simulink model "SIMULINK_flexible_joint"  (R2024b)
settings: Solver=ode45  StartTime=0.0  StopTime=100  RelTol=1e-3  EnableMultiTasking=on
undefined symbols (not defined in the file): cix1, cix2, cix3, cix4, g, hcm, Jh, Jl, Kg, Km, Ks, Kz, Kzi, m, pert, Rm
libraries: simulink x1
settings Model: Creator=AP  LastModifiedBy=J Ferb
settings SolverCC: AlgebraicLoopSolver=TrustRegion
settings DataIOCC: LimitDataPoints=on  SaveFormat=Array  SignalLoggingSaveFormat=ModelDataLogs  ReturnWorkspaceOutputs=off
settings OptimizationCC: ExpressionDepthLimit=2147483647  InitFltsAndDblsToZero=on  LifeSpan=inf
settings DebuggingCC: SaveWithParameterizedLinksMsg=none  UnderspecifiedInitializationDetection=Classic  MergeDetectMultiDrivingBlocksExec=none  FcnCallInpInsideContextMsg=warning  UnconnectedInputMsg=warning  UnconnectedOutputMsg=warning  UnconnectedLineMsg=warning  StateNameClashWarn=warning  SFUnexpectedBacktrackingDiag=warning  SFNoUnconditionalDefaultTransitionDiag=warning  SFExecutionAtInitializationDiag=none  ArithmeticOperatorsInVariantConditions=warning
settings HardwareCC: ProdBitPerPointer=32  ProdBitPerSizeT=32  ProdBitPerPtrDiffT=32  ProdLargestAtomicFloat=None  ProdIntDivRoundTo=Undefined  ProdEndianess=Unspecified  ProdWordSize=32  ProdHWDeviceType=32-bit Generic
settings ModelReferenceCC: EnableRefExpFcnMdlSchedulingChecks=on  PropagateSignalLabelsOutOfModel=off
settings SFSimCC: SimParseCustomCode=off
settings RTWCC: GPUComputeCapability=3.5
settings CodeAppCC: StateflowObjectComments=on
settings GRTTargetCC: TargetFcnLib=ansi_tfl_tmw.mat  TargetLangStandard=C89/C90 (ANSI)  CombineOutputUpdateFcns=off  GRTInterface=on
settings ConfigComp: CovMetricSettings=dw  CovSaveCumulativeToWorkspaceVar=on  CovSaveSingleToWorkspaceVar=on

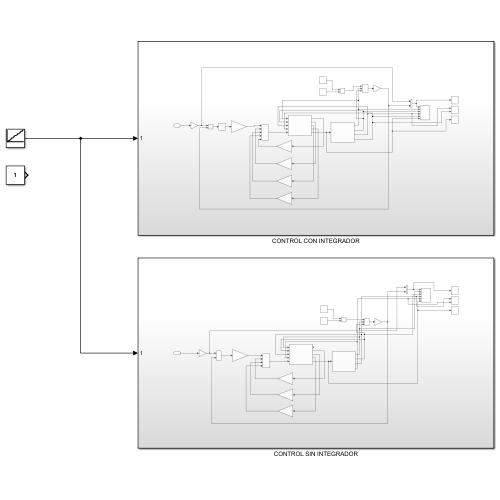
[thumbnail: Simulink's stored preview of the top-level diagram]
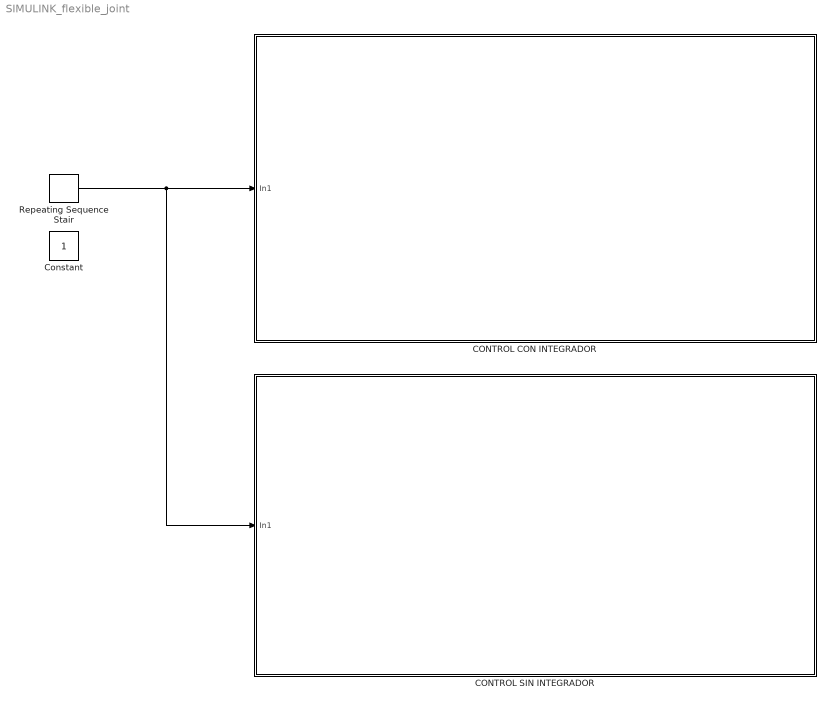
== system SIMULINK_flexible_joint ==
  CONTROL CON INTEGRADOR : Subsystem
  CONTROL SIN INTEGRADOR : Subsystem
  Constant : Constant
  Repeating Sequence Stair : simulink/Sources/Repeating Sequence Stair  OutValues=[0 0.02 0.04 0.06 0.08 0.1 0.12 0.14 0.16 0.18 0.2].'*1  tsamp=4  OutMin=[]  OutMax=[]  OutDataTypeStr=float('double')  OutputDataTypeScalingMode=Specify via dialog  OutDataType=float('double')  ConRadixGroup=Best Precision: Vector-wise  OutScaling=2^-12
  wires:
  Repeating Sequence Stair/1 -> CONTROL SIN INTEGRADOR/1(In1), CONTROL CON INTEGRADOR/1(In1)

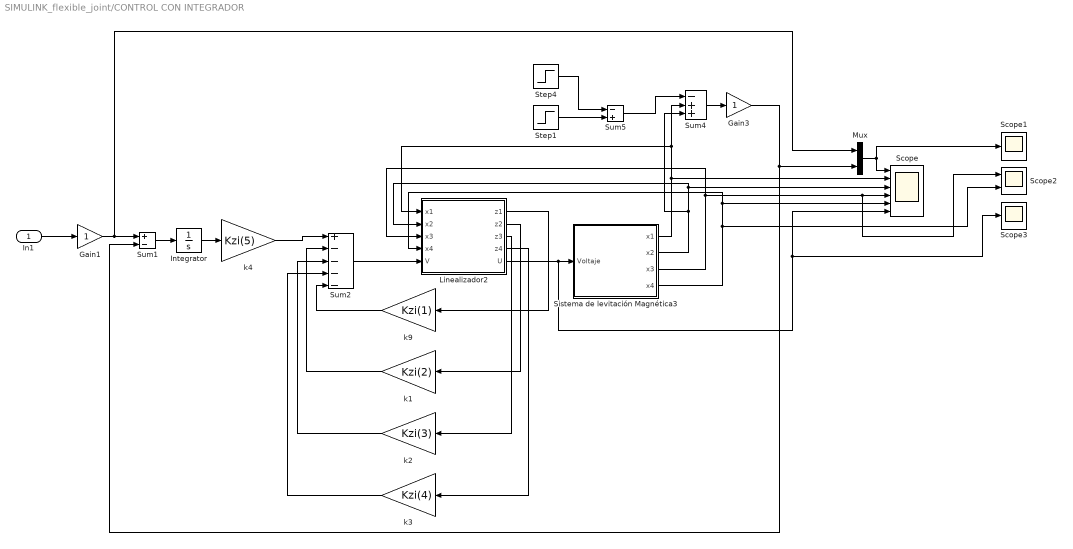
== system SIMULINK_flexible_joint/CONTROL CON INTEGRADOR ==
  In1 : Inport
  Gain1 : Gain
  Gain3 : Gain
  Integrator : Integrator
  Linealizador2 : Subsystem
  Mux : Mux  Inputs=2
  Scope : Scope  NumInputPorts=6
  Scope1 : Scope
  Scope2 : Scope  NumInputPorts=2
  Scope3 : Scope
  Sistema de levitación Magnética3 : Subsystem
  Step1 : Step  Time=5  After=pert  SampleTime=0
  Step4 : Step  Time=5.1  After=pert  SampleTime=0
  Sum1 : Sum  Inputs=+-
  Sum2 : Sum  Inputs=+----
  Sum4 : Sum  Inputs=-++
  Sum5 : Sum  Inputs=-+
  k1 : Gain  Gain=Kzi(2)
  k2 : Gain  Gain=Kzi(3)
  k3 : Gain  Gain=Kzi(4)
  k4 : Gain  Gain=Kzi(5)
  k9 : Gain  Gain=Kzi(1)
  wires:
  Sistema de levitación Magnética3/4(x4) -> Scope/5, Linealizador2/4(x4), Scope2/2
  Linealizador2/1(z1) -> k9/1
  Sum4/1 -> Gain3/1
  Sistema de levitación Magnética3/1(x1) -> Sum4/2, Linealizador2/1(x1), Scope/2
  k3/1 -> Sum2/4
  Linealizador2/4(z4) -> k3/1
  k1/1 -> Sum2/2
  k2/1 -> Sum2/3
  In1/1 -> Gain1/1
  Linealizador2/3(z3) -> k2/1
  Gain1/1 -> Mux/1, Sum1/1
  Linealizador2/5(U) -> Sistema de levitación Magnética3/1(Voltaje), Scope3/1, Scope/6
  Mux/1 -> Scope1/1, Scope/1
  Sum5/1 -> Sum4/1
  Sum1/1 -> Integrator/1
  Step1/1 -> Sum5/2
  k9/1 -> Sum2/5
  Step4/1 -> Sum5/1
  Sistema de levitación Magnética3/3(x3) -> Scope2/1, Scope/4, Linealizador2/3(x3)
  Integrator/1 -> k4/1
  Sum2/1 -> Linealizador2/5(V)
  k4/1 -> Sum2/1
  Sistema de levitación Magnética3/2(x2) -> Sum4/3, Scope/3, Linealizador2/2(x2)
  Gain3/1 -> Mux/2, Sum1/2
  Linealizador2/2(z2) -> k1/1

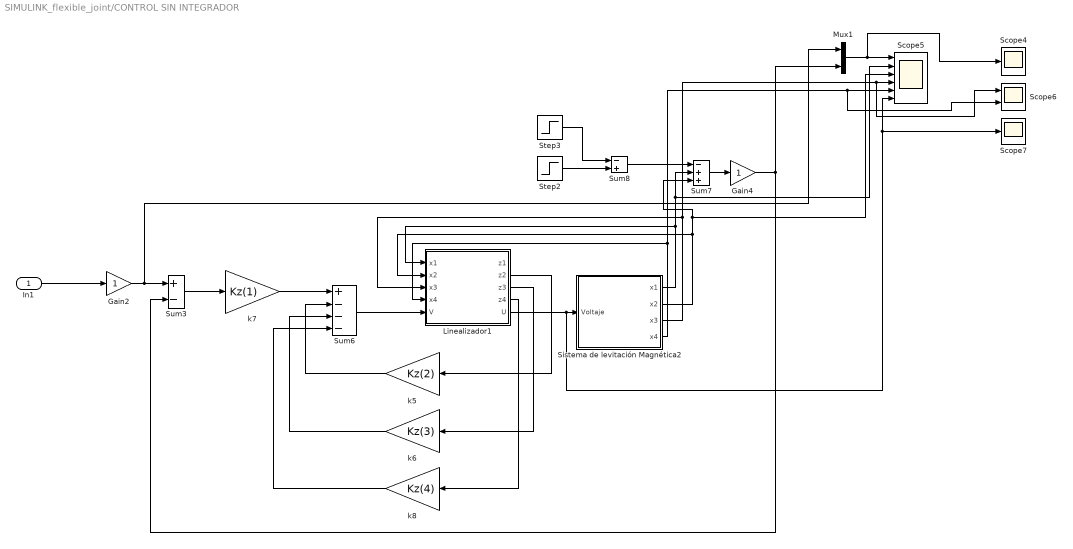
== system SIMULINK_flexible_joint/CONTROL SIN INTEGRADOR ==
  In1 : Inport
  Gain2 : Gain
  Gain4 : Gain
  Linealizador1 : Subsystem
  Mux1 : Mux  Inputs=2
  Scope4 : Scope
  Scope5 : Scope  NumInputPorts=6
  Scope6 : Scope  NumInputPorts=2
  Scope7 : Scope
  Sistema de levitación Magnética2 : Subsystem
  Step2 : Step  Time=5  After=pert  SampleTime=0
  Step3 : Step  Time=5.1  After=pert  SampleTime=0
  Sum3 : Sum  Inputs=+-
  Sum6 : Sum  Inputs=+---
  Sum7 : Sum  Inputs=-++
  Sum8 : Sum  Inputs=-+
  k5 : Gain  Gain=Kz(2)
  k6 : Gain  Gain=Kz(3)
  k7 : Gain  Gain=Kz(1)
  k8 : Gain  Gain=Kz(4)
  wires:
  Linealizador1/2(z2) -> k5/1
  k7/1 -> Sum6/1
  k6/1 -> Sum6/3
  Linealizador1/3(z3) -> k6/1
  Step3/1 -> Sum8/1
  Sistema de levitación Magnética2/4(x4) -> Linealizador1/4(x4), Scope6/2, Scope5/5
  Gain2/1 -> Mux1/1, Sum3/1
  k8/1 -> Sum6/4
  Linealizador1/5(U) -> Scope7/1, Scope5/6, Sistema de levitación Magnética2/1(Voltaje)
  Gain4/1 -> Mux1/2, Sum3/2
  Sistema de levitación Magnética2/1(x1) -> Sum7/2, Scope5/2, Linealizador1/1(x1)
  Sum8/1 -> Sum7/1
  Mux1/1 -> Scope4/1, Scope5/1
  Sum3/1 -> k7/1
  Sistema de levitación Magnética2/3(x3) -> Linealizador1/3(x3), Scope5/4, Scope6/1
  In1/1 -> Gain2/1
  Sistema de levitación Magnética2/2(x2) -> Scope5/3, Sum7/3, Linealizador1/2(x2)
  Sum6/1 -> Linealizador1/5(V)
  Step2/1 -> Sum8/2
  Linealizador1/4(z4) -> k8/1
  Sum7/1 -> Gain4/1
  k5/1 -> Sum6/2

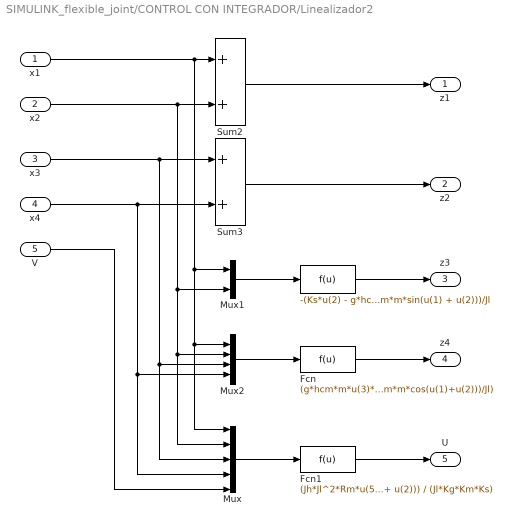
== system SIMULINK_flexible_joint/CONTROL CON INTEGRADOR/Linealizador2 ==
  x1 : Inport
  x2 : Inport  Port=2
  x3 : Inport  Port=3
  x4 : Inport  Port=4
  V : Inport  Port=5
  " " : Fcn  Expr=-(Ks*u(2) - g*hcm*m*sin(u(1) + u(2)))/Jl
  Fcn : Fcn  Expr=(g*hcm*m*u(3)*cos(u(1)+u(2)))/Jl - u(4)*((Ks/Jl) - (g*hcm*m*cos(u(1)+u(2)))/Jl)
  Fcn1 : Fcn  Expr=|
      | (Jh*Jl^2*Rm*u(5) - Jh*Ks^2*Rm*u(2) - Jl*Ks^2*Rm*u(2) + Jl*Kg^2*Km^2*Ks*u(3) 
      | - (Jh*Rm*g^2*hcm^2*m^2*sin(2*u(1) + 2*u(2)))/2 + Jh*Ks*Rm*g*hcm*m*sin(u(1) + u(2)) 
      | + Jh*Jl*Rm*g*hcm*m*u(3)^2*sin(u(1) + u(2)) + Jh*Jl*Rm*g*hcm*m*u(4)^2*sin(u(1) + u(2)) 
      | + Jh*Ks*Rm*g*hcm*m*u(2)*cos(u(1) + u(2)) + 2*Jh*Jl*Rm*g*hcm*m*u(3)*u(4)*sin(u(1) + u(2))) / (Jl*Kg*Km*Ks)
  Mux : Mux  Inputs=5
  Mux1 : Mux  Inputs=2
  Mux2 : Mux
  Sum2 : Sum
  Sum3 : Sum
  z1 : Outport
  z2 : Outport  Port=2
  z3 : Outport  Port=3
  z4 : Outport  Port=4
  U : Outport  Port=5
  wires:
  " "/1 -> z3/1
  Sum3/1 -> z2/1
  Mux1/1 -> " "/1
  x4/1 -> Mux2/4, Mux/4, Sum3/2
  Sum2/1 -> z1/1
  x2/1 -> Mux/2, Mux2/2, Mux1/2, Sum2/2
  Fcn1/1 -> U/1
  x1/1 -> Mux/1, Mux2/1, Mux1/1, Sum2/1
  x3/1 -> Mux/3, Mux2/3, Sum3/1
  Mux2/1 -> Fcn/1
  Mux/1 -> Fcn1/1
  Fcn/1 -> z4/1
  V/1 -> Mux/5

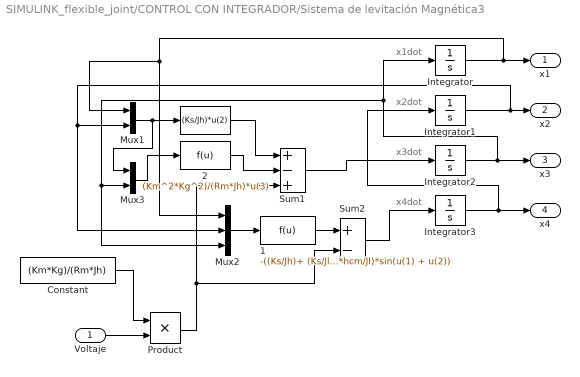
== system SIMULINK_flexible_joint/CONTROL CON INTEGRADOR/Sistema de levitación Magnética3 ==
  note: x1dot
  note: x2dot
  note: x3dot
  note: x4dot
  Voltaje : Inport
  " " : Fcn  Expr=(Ks/Jh)*u(2)
  " 1" : Fcn  Expr=-((Ks/Jh)+ (Ks/Jl))*u(2) + (Km^2*Kg^2)/(Rm*Jh)*u(3) + (m*g*hcm/Jl)*sin(u(1) + u(2))
  " 2" : Fcn  Expr=(Km^2*Kg^2)/(Rm*Jh)*u(3)
  Constant : Constant  Value=(Km*Kg)/(Rm*Jh)
  Integrator : Integrator  InitialCondition=cix1
  Integrator1 : Integrator  InitialCondition=cix2
  Integrator2 : Integrator  InitialCondition=cix3
  Integrator3 : Integrator  InitialCondition=cix4
  Mux1 : Mux  Inputs=2
  Mux2 : Mux  Inputs=3
  Mux3 : Mux  Inputs=2
  Product : Product  RndMeth=Zero
  Sum1 : Sum  Inputs=+-+
  Sum2 : Sum  Inputs=+-
  x1 : Outport
  x2 : Outport  Port=2
  x3 : Outport  Port=3
  x4 : Outport  Port=4
  wires:
  Integrator/1 -> Mux1/1, Mux2/1, x1/1
  Integrator1/1 -> Mux1/2, Mux2/2, x2/1
  Integrator2/1 -> Integrator/1, Mux3/2, Mux2/3, x3/1
  Integrator3/1 -> Integrator1/1, x4/1
  " "/1 -> Sum1/1
  Sum1/1 -> Integrator2/1
  Voltaje/1 -> Product/2
  Constant/1 -> Product/1
  Product/1 -> Sum1/3, Sum2/2
  Mux2/1 -> " 1"/1
  " 1"/1 -> Sum2/1
  Sum2/1 -> Integrator3/1
  " 2"/1 -> Sum1/2
  Mux1/1 -> Mux3/1, " "/1
  Mux3/1 -> " 2"/1

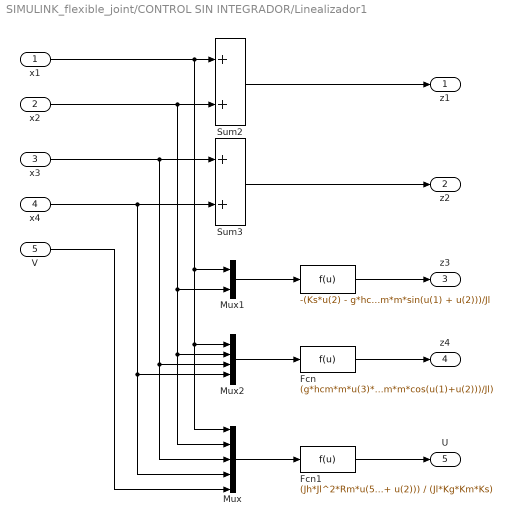
== system SIMULINK_flexible_joint/CONTROL SIN INTEGRADOR/Linealizador1 ==
  x1 : Inport
  x2 : Inport  Port=2
  x3 : Inport  Port=3
  x4 : Inport  Port=4
  V : Inport  Port=5
  " " : Fcn  Expr=-(Ks*u(2) - g*hcm*m*sin(u(1) + u(2)))/Jl
  Fcn : Fcn  Expr=(g*hcm*m*u(3)*cos(u(1)+u(2)))/Jl - u(4)*((Ks/Jl) - (g*hcm*m*cos(u(1)+u(2)))/Jl)
  Fcn1 : Fcn  Expr=|
      | (Jh*Jl^2*Rm*u(5) - Jh*Ks^2*Rm*u(2) - Jl*Ks^2*Rm*u(2) + Jl*Kg^2*Km^2*Ks*u(3) 
      | - (Jh*Rm*g^2*hcm^2*m^2*sin(2*u(1) + 2*u(2)))/2 + Jh*Ks*Rm*g*hcm*m*sin(u(1) + u(2)) 
      | + Jh*Jl*Rm*g*hcm*m*u(3)^2*sin(u(1) + u(2)) + Jh*Jl*Rm*g*hcm*m*u(4)^2*sin(u(1) + u(2)) 
      | + Jh*Ks*Rm*g*hcm*m*u(2)*cos(u(1) + u(2)) + 2*Jh*Jl*Rm*g*hcm*m*u(3)*u(4)*sin(u(1) + u(2))) / (Jl*Kg*Km*Ks)
  Mux : Mux  Inputs=5
  Mux1 : Mux  Inputs=2
  Mux2 : Mux
  Sum2 : Sum
  Sum3 : Sum
  z1 : Outport
  z2 : Outport  Port=2
  z3 : Outport  Port=3
  z4 : Outport  Port=4
  U : Outport  Port=5
  wires:
  " "/1 -> z3/1
  Sum3/1 -> z2/1
  Mux1/1 -> " "/1
  x4/1 -> Mux2/4, Mux/4, Sum3/2
  Sum2/1 -> z1/1
  x2/1 -> Mux/2, Mux2/2, Mux1/2, Sum2/2
  Fcn1/1 -> U/1
  x1/1 -> Mux/1, Mux2/1, Mux1/1, Sum2/1
  x3/1 -> Mux/3, Mux2/3, Sum3/1
  Mux2/1 -> Fcn/1
  Mux/1 -> Fcn1/1
  Fcn/1 -> z4/1
  V/1 -> Mux/5

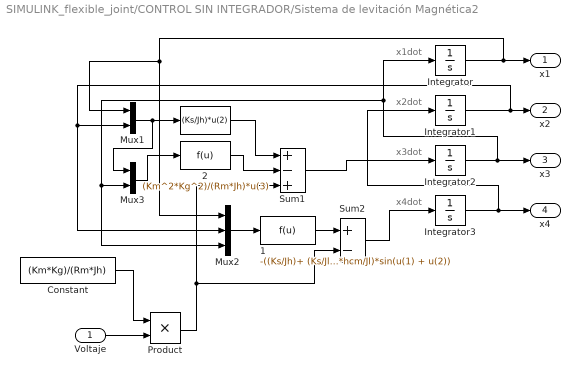
== system SIMULINK_flexible_joint/CONTROL SIN INTEGRADOR/Sistema de levitación Magnética2 ==
  note: x1dot
  note: x2dot
  note: x3dot
  note: x4dot
  Voltaje : Inport
  " " : Fcn  Expr=(Ks/Jh)*u(2)
  " 1" : Fcn  Expr=-((Ks/Jh)+ (Ks/Jl))*u(2) + (Km^2*Kg^2)/(Rm*Jh)*u(3) + (m*g*hcm/Jl)*sin(u(1) + u(2))
  " 2" : Fcn  Expr=(Km^2*Kg^2)/(Rm*Jh)*u(3)
  Constant : Constant  Value=(Km*Kg)/(Rm*Jh)
  Integrator : Integrator  InitialCondition=cix1
  Integrator1 : Integrator  InitialCondition=cix2
  Integrator2 : Integrator  InitialCondition=cix3
  Integrator3 : Integrator  InitialCondition=cix4
  Mux1 : Mux  Inputs=2
  Mux2 : Mux  Inputs=3
  Mux3 : Mux  Inputs=2
  Product : Product  RndMeth=Zero
  Sum1 : Sum  Inputs=+-+
  Sum2 : Sum  Inputs=+-
  x1 : Outport
  x2 : Outport  Port=2
  x3 : Outport  Port=3
  x4 : Outport  Port=4
  wires:
  Integrator/1 -> Mux1/1, Mux2/1, x1/1
  Integrator1/1 -> Mux1/2, Mux2/2, x2/1
  Integrator2/1 -> Integrator/1, Mux3/2, Mux2/3, x3/1
  Integrator3/1 -> Integrator1/1, x4/1
  " "/1 -> Sum1/1
  Sum1/1 -> Integrator2/1
  Voltaje/1 -> Product/2
  Constant/1 -> Product/1
  Product/1 -> Sum1/3, Sum2/2
  Mux2/1 -> " 1"/1
  " 1"/1 -> Sum2/1
  Sum2/1 -> Integrator3/1
  " 2"/1 -> Sum1/2
  Mux1/1 -> Mux3/1, " "/1
  Mux3/1 -> " 2"/1
